simulink model "StorqueV2"  (Simulink 7.5)
settings: Solver=ode45  StartTime=0.0  StopTime=10.0  RelTol=1e-3
undefined symbols (not defined in the file or in its folder): armLength, g, Ixx, Iyy, Izz, KdPhi, KdPsi, KdTheta, KiPhi, KiPsi, KiTheta, KpPhi, KpPsi, KpTheta, mass, PWMMax, PWMMin, PWMPerThrust, tau1, tau2, tau3, tau4
settings Model: Creator=ianohara  LastModifiedBy=ianohara

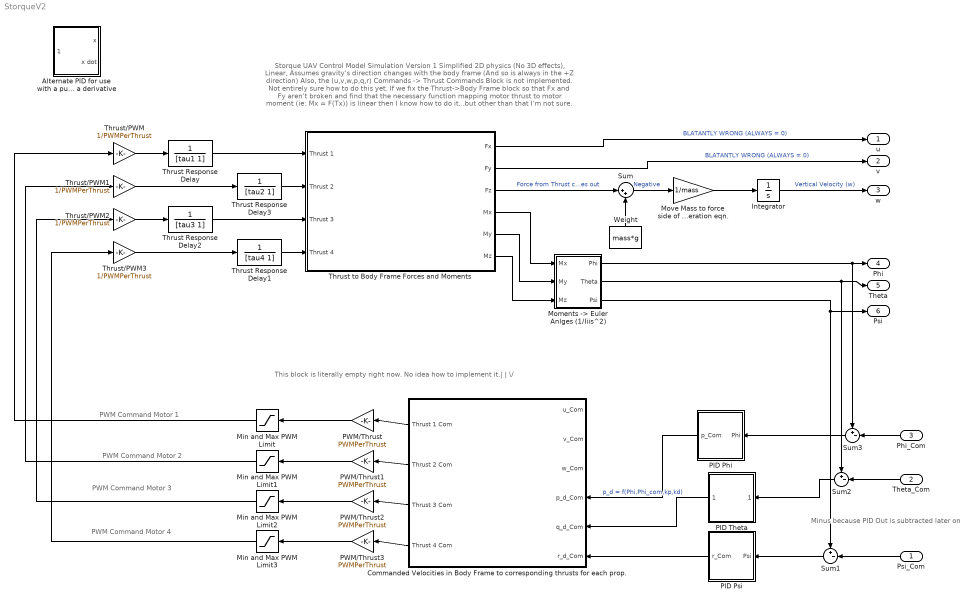
== system StorqueV2 ==
  note: PWM Command Motor 1
  note: PWM Command Motor 2
  note: PWM Command Motor 3
  note: PWM Command Motor 4
  note: This block is literally empty right now.
      | No idea how to implement it.|
      |                                               |
      |                                                \/
  note: Storque UAV Control Model Simulation Version 1
      | Simplified 2D physics (No 3D effects), Linear, Assumes gravity's direction changes with
      | the body frame (And so is always in the +Z direction)
      |
      | Also, the (u,v,w,p,q,r) Commands -> Thrust Commands Block is not implemented.
      | Not entirely sure how to do this yet.  If we fix the Thrust->Body Frame block so that
      | Fx and Fy aren't broken and find that the necessary function mapping motor thrust to motor
      | moment (ie: Mx = F(Tx)) is linear then I know how to do it...but other than that I'm not sure.
  note: Minus because PID
      | Out is subtracted later on
  Psi_Com : Inport  OutDataType=fixdt(1, 16)  OutScaling=2^0
  Theta_Com : Inport  Port=2  OutDataType=fixdt(1, 16)  OutScaling=2^0
  Phi_Com : Inport  Port=3  OutDataType=fixdt(1, 16)  OutScaling=2^0
  Alternate PID for use with a pure rate signal instead of taking a derivative : Subsystem
  Commanded Velocities in Body Frame to corresponding thrusts for each prop. : Subsystem
  Integrator : Integrator
  Min and Max PWM Limit{,1..3} (4 alike) : Saturate  UpperLimit=PWMMax  LowerLimit=PWMMin  OutDataType=fixdt(1, 16)  OutScaling=2^0
  "Moments -> Euler Anlges (1/Iiis^2)" : Subsystem
  Move Mass to force side of acceleration eqn. : Gain  Gain=1/mass  ParameterDataType=fixdt(1, 16)  ParameterScaling=2^0  OutDataType=fixdt(1, 16)  OutScaling=2^0
  PID Phi : Subsystem
  PID Psi : Subsystem
  PID Theta : Subsystem
  PWM/Thrust{,1..3} (4 alike) : Gain  Gain=PWMPerThrust  ParameterDataType=fixdt(1, 16)  ParameterScaling=2^0  OutDataType=fixdt(1, 16)  OutScaling=2^0
  Sum : Sum  Inputs=|++  OutDataType=fixdt(1, 16)  OutScaling=2^0
  Sum1 : Sum  Inputs=+-|  OutDataType=fixdt(1, 16)  OutScaling=2^0
  Sum2 : Sum  Inputs=+-|  OutDataType=fixdt(1, 16)  OutScaling=2^0
  Sum3 : Sum  Inputs=+-|  OutDataType=fixdt(1, 16)  OutScaling=2^0
  Thrust Response Delay : TransferFcn  Denominator=[tau1 1]
  Thrust Response Delay1 : TransferFcn  Denominator=[tau4 1]
  Thrust Response Delay2 : TransferFcn  Denominator=[tau3 1]
  Thrust Response Delay3 : TransferFcn  Denominator=[tau2 1]
  Thrust to Body Frame Forces and Moments : Subsystem  Description=This simulates the body frame reactions of the Storque due to the application of a particular thrust at each of the 4 props.
  Thrust/PWM{,1..3} (4 alike) : Gain  Gain=1/PWMPerThrust  ParameterDataType=fixdt(1, 16)  ParameterScaling=2^0  OutDataType=fixdt(1, 16)  OutScaling=2^0
  Weight : Constant  Value=mass*g  OutDataType=fixdt(1, 16)  OutScaling=2^0
  u : Outport  OutDataType=fixdt(1, 16)  OutScaling=2^0
  v : Outport  Port=2  OutDataType=fixdt(1, 16)  OutScaling=2^0
  w : Outport  Port=3  OutDataType=fixdt(1, 16)  OutScaling=2^0
  Phi : Outport  Port=4  OutDataType=fixdt(1, 16)  OutScaling=2^0
  Theta : Outport  Port=5  OutDataType=fixdt(1, 16)  OutScaling=2^0
  Psi : Outport  Port=6  OutDataType=fixdt(1, 16)  OutScaling=2^0
  wires:
  Thrust to Body Frame Forces and Moments/3(Fz) -> Sum/1  "Force from Thrust comes out                 Negative"
  Weight/1 -> Sum/2
  Sum/1 -> Move Mass to force side of acceleration eqn./1
  Move Mass to force side of acceleration eqn./1 -> Integrator/1
  Integrator/1 -> w/1  "Vertical Velocity (w)"
  Thrust to Body Frame Forces and Moments/6(Mz) -> "Moments -> Euler Anlges (1/Iiis^2)"/3(Mz)
  Thrust to Body Frame Forces and Moments/5(My) -> "Moments -> Euler Anlges (1/Iiis^2)"/2(My)
  Thrust to Body Frame Forces and Moments/4(Mx) -> "Moments -> Euler Anlges (1/Iiis^2)"/1(Mx)
  Thrust to Body Frame Forces and Moments/1(Fx) -> u/1  "BLATANTLY WRONG (ALWAYS = 0)"
  Thrust to Body Frame Forces and Moments/2(Fy) -> v/1  "BLATANTLY WRONG (ALWAYS = 0)"
  "Moments -> Euler Anlges (1/Iiis^2)"/1(Phi) -> Phi/1, Sum3/1
  "Moments -> Euler Anlges (1/Iiis^2)"/2(Theta) -> Theta/1, Sum2/1
  "Moments -> Euler Anlges (1/Iiis^2)"/3(Psi) -> Sum1/1, Psi/1
  Sum1/1 -> PID Psi/1(Psi)
  Sum2/1 -> PID Theta/1(Theta)
  Sum3/1 -> PID Phi/1(Phi)
  Psi_Com/1 -> Sum1/2
  Theta_Com/1 -> Sum2/2
  Phi_Com/1 -> Sum3/2
  Thrust Response Delay/1 -> Thrust to Body Frame Forces and Moments/1(Thrust 1)
  Thrust Response Delay3/1 -> Thrust to Body Frame Forces and Moments/2(Thrust 2)
  Thrust Response Delay2/1 -> Thrust to Body Frame Forces and Moments/3(Thrust 3)
  Thrust Response Delay1/1 -> Thrust to Body Frame Forces and Moments/4(Thrust 4)
  PID Psi/1(r_Com) -> Commanded Velocities in Body Frame to corresponding thrusts for each prop./6(r_d_Com)
  PID Theta/1(q_Com) -> Commanded Velocities in Body Frame to corresponding thrusts for each prop./5(q_d_Com)
  PID Phi/1(p_Com) -> Commanded Velocities in Body Frame to corresponding thrusts for each prop./4(p_d_Com)  "p_d = f(Phi,Phi_com,kp,kd)"
  Commanded Velocities in Body Frame to corresponding thrusts for each prop./1(Thrust 1 Com) -> PWM/Thrust/1
  Commanded Velocities in Body Frame to corresponding thrusts for each prop./2(Thrust 2 Com) -> PWM/Thrust1/1
  Commanded Velocities in Body Frame to corresponding thrusts for each prop./3(Thrust 3 Com) -> PWM/Thrust2/1
  Commanded Velocities in Body Frame to corresponding thrusts for each prop./4(Thrust 4 Com) -> PWM/Thrust3/1
  PWM/Thrust/1 -> Min and Max PWM Limit/1
  PWM/Thrust1/1 -> Min and Max PWM Limit1/1
  PWM/Thrust2/1 -> Min and Max PWM Limit2/1
  PWM/Thrust3/1 -> Min and Max PWM Limit3/1
  Min and Max PWM Limit/1 -> Thrust/PWM/1
  Min and Max PWM Limit1/1 -> Thrust/PWM1/1
  Min and Max PWM Limit2/1 -> Thrust/PWM2/1
  Min and Max PWM Limit3/1 -> Thrust/PWM3/1
  Thrust/PWM3/1 -> Thrust Response Delay1/1
  Thrust/PWM2/1 -> Thrust Response Delay2/1
  Thrust/PWM1/1 -> Thrust Response Delay3/1
  Thrust/PWM/1 -> Thrust Response Delay/1

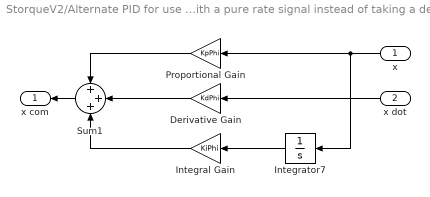
== system StorqueV2/Alternate PID for use with a pure rate signal instead of taking a derivative ==
  x : Inport  OutDataType=fixdt(1, 16)  OutScaling=2^0
  x dot : Inport  Port=2  OutDataType=fixdt(1, 16)  OutScaling=2^0
  Derivative Gain : Gain  Gain=KdPhi  ParameterDataType=fixdt(1, 16)  ParameterScaling=2^0  OutDataType=fixdt(1, 16)  OutScaling=2^0
  Integral Gain : Gain  Gain=KiPhi  ParameterDataType=fixdt(1, 16)  ParameterScaling=2^0  OutDataType=fixdt(1, 16)  OutScaling=2^0
  Integrator7 : Integrator
  Proportional Gain : Gain  Gain=KpPhi  ParameterDataType=fixdt(1, 16)  ParameterScaling=2^0  OutDataType=fixdt(1, 16)  OutScaling=2^0
  Sum1 : Sum  Inputs=+++  OutDataType=fixdt(1, 16)  OutScaling=2^0
  x com : Outport
  wires:
  Integral Gain/1 -> Sum1/3
  Derivative Gain/1 -> Sum1/2
  Proportional Gain/1 -> Sum1/1
  x dot/1 -> Derivative Gain/1
  Integrator7/1 -> Integral Gain/1
  Sum1/1 -> x com/1
  x/1 -> Proportional Gain/1, Integrator7/1

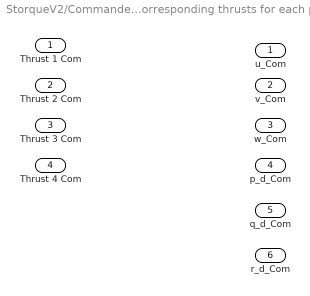
== system StorqueV2/Commanded Velocities in Body Frame to corresponding thrusts for each prop. ==
  u_Com : Inport  OutDataType=fixdt(1, 16)  OutScaling=2^0
  v_Com : Inport  Port=2  OutDataType=fixdt(1, 16)  OutScaling=2^0
  w_Com : Inport  Port=3  OutDataType=fixdt(1, 16)  OutScaling=2^0
  p_d_Com : Inport  Port=4  OutDataType=fixdt(1, 16)  OutScaling=2^0
  q_d_Com : Inport  Port=5  OutDataType=fixdt(1, 16)  OutScaling=2^0
  r_d_Com : Inport  Port=6  OutDataType=fixdt(1, 16)  OutScaling=2^0
  Thrust 1 Com : Outport  OutDataType=fixdt(1, 16)  OutScaling=2^0
  Thrust 2 Com : Outport  Port=2  OutDataType=fixdt(1, 16)  OutScaling=2^0
  Thrust 3 Com : Outport  Port=3  OutDataType=fixdt(1, 16)  OutScaling=2^0
  Thrust 4 Com : Outport  Port=4  OutDataType=fixdt(1, 16)  OutScaling=2^0

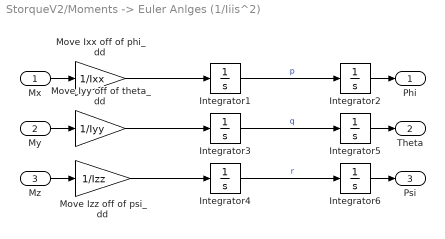
== system StorqueV2/Moments -> Euler Anlges (1/Iiis^2) ==
  Mx : Inport
  My : Inport  Port=2
  Mz : Inport  Port=3
  Integrator{1..6} (6 alike) : Integrator
  Move Ixx off of phi_dd : Gain  Gain=1/Ixx  ParameterDataType=fixdt(1, 16)  ParameterScaling=2^0  OutDataType=fixdt(1, 16)  OutScaling=2^0
  Move Iyy off of theta_dd : Gain  Gain=1/Iyy  ParameterDataType=fixdt(1, 16)  ParameterScaling=2^0  OutDataType=fixdt(1, 16)  OutScaling=2^0
  Move Izz off of psi_dd : Gain  Gain=1/Izz  ParameterDataType=fixdt(1, 16)  ParameterScaling=2^0  OutDataType=fixdt(1, 16)  OutScaling=2^0
  Phi : Outport
  Theta : Outport  Port=2
  Psi : Outport  Port=3
  wires:
  Move Ixx off of phi_dd/1 -> Integrator1/1
  Integrator1/1 -> Integrator2/1  "p"
  Move Iyy off of theta_dd/1 -> Integrator3/1
  Integrator3/1 -> Integrator5/1  "q"
  Move Izz off of psi_dd/1 -> Integrator4/1
  Integrator4/1 -> Integrator6/1  "r"
  Integrator2/1 -> Phi/1
  Mx/1 -> Move Ixx off of phi_dd/1
  Integrator5/1 -> Theta/1
  My/1 -> Move Iyy off of theta_dd/1
  Integrator6/1 -> Psi/1
  Mz/1 -> Move Izz off of psi_dd/1

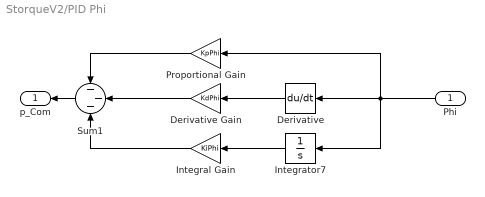
== system StorqueV2/PID Phi ==
  Phi : Inport  OutDataType=fixdt(1, 16)  OutScaling=2^0
  Derivative : Derivative
  Derivative Gain : Gain  Gain=KdPhi  ParameterDataType=fixdt(1, 16)  ParameterScaling=2^0  OutDataType=fixdt(1, 16)  OutScaling=2^0
  Integral Gain : Gain  Gain=KiPhi  ParameterDataType=fixdt(1, 16)  ParameterScaling=2^0  OutDataType=fixdt(1, 16)  OutScaling=2^0
  Integrator7 : Integrator
  Proportional Gain : Gain  Gain=KpPhi  ParameterDataType=fixdt(1, 16)  ParameterScaling=2^0  OutDataType=fixdt(1, 16)  OutScaling=2^0
  Sum1 : Sum  Inputs=---  OutDataType=fixdt(1, 16)  OutScaling=2^0
  p_Com : Outport
  wires:
  Integral Gain/1 -> Sum1/3
  Derivative Gain/1 -> Sum1/2
  Proportional Gain/1 -> Sum1/1
  Derivative/1 -> Derivative Gain/1
  Integrator7/1 -> Integral Gain/1
  Phi/1 -> Derivative/1, Proportional Gain/1, Integrator7/1
  Sum1/1 -> p_Com/1

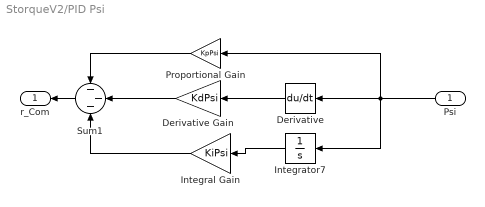
== system StorqueV2/PID Psi ==
  Psi : Inport  OutDataType=fixdt(1, 16)  OutScaling=2^0
  Derivative : Derivative
  Derivative Gain : Gain  Gain=KdPsi  ParameterDataType=fixdt(1, 16)  ParameterScaling=2^0  OutDataType=fixdt(1, 16)  OutScaling=2^0
  Integral Gain : Gain  Gain=KiPsi  ParameterDataType=fixdt(1, 16)  ParameterScaling=2^0  OutDataType=fixdt(1, 16)  OutScaling=2^0
  Integrator7 : Integrator
  Proportional Gain : Gain  Gain=KpPsi  ParameterDataType=fixdt(1, 16)  ParameterScaling=2^0  OutDataType=fixdt(1, 16)  OutScaling=2^0
  Sum1 : Sum  Inputs=---  OutDataType=fixdt(1, 16)  OutScaling=2^0
  r_Com : Outport
  wires:
  Integral Gain/1 -> Sum1/3
  Derivative Gain/1 -> Sum1/2
  Proportional Gain/1 -> Sum1/1
  Derivative/1 -> Derivative Gain/1
  Integrator7/1 -> Integral Gain/1
  Psi/1 -> Derivative/1, Proportional Gain/1, Integrator7/1
  Sum1/1 -> r_Com/1

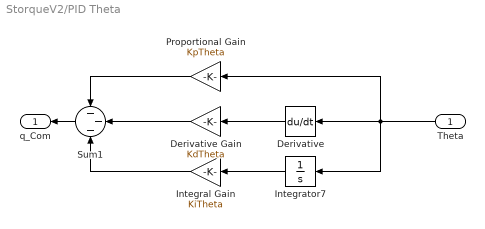
== system StorqueV2/PID Theta ==
  Theta : Inport  OutDataType=fixdt(1, 16)  OutScaling=2^0
  Derivative : Derivative
  Derivative Gain : Gain  Gain=KdTheta  ParameterDataType=fixdt(1, 16)  ParameterScaling=2^0  OutDataType=fixdt(1, 16)  OutScaling=2^0
  Integral Gain : Gain  Gain=KiTheta  ParameterDataType=fixdt(1, 16)  ParameterScaling=2^0  OutDataType=fixdt(1, 16)  OutScaling=2^0
  Integrator7 : Integrator
  Proportional Gain : Gain  Gain=KpTheta  ParameterDataType=fixdt(1, 16)  ParameterScaling=2^0  OutDataType=fixdt(1, 16)  OutScaling=2^0
  Sum1 : Sum  Inputs=---  OutDataType=fixdt(1, 16)  OutScaling=2^0
  q_Com : Outport
  wires:
  Integral Gain/1 -> Sum1/3
  Derivative Gain/1 -> Sum1/2
  Proportional Gain/1 -> Sum1/1
  Derivative/1 -> Derivative Gain/1
  Integrator7/1 -> Integral Gain/1
  Theta/1 -> Derivative/1, Proportional Gain/1, Integrator7/1
  Sum1/1 -> q_Com/1

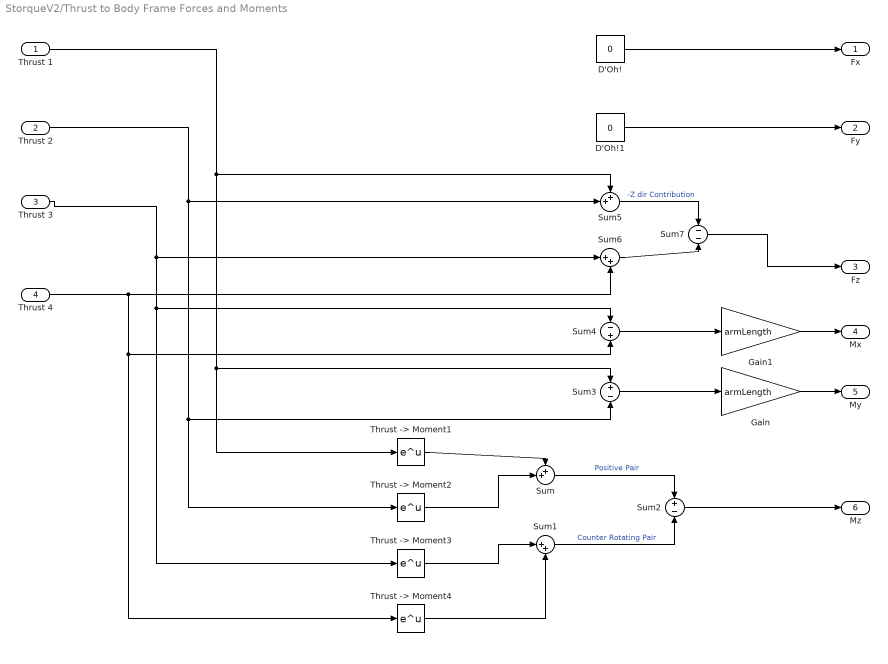
== system StorqueV2/Thrust to Body Frame Forces and Moments ==
  Thrust 1 : Inport  OutDataType=fixdt(1, 16)  OutScaling=2^0
  Thrust 2 : Inport  Port=2  OutDataType=fixdt(1, 16)  OutScaling=2^0
  Thrust 3 : Inport  Port=3  OutDataType=fixdt(1, 16)  OutScaling=2^0
  Thrust 4 : Inport  Port=4  OutDataType=fixdt(1, 16)  OutScaling=2^0
  D'Oh! : Constant  Value=0  OutDataType=fixdt(1, 16)  OutScaling=2^0
  D'Oh!1 : Constant  Value=0  OutDataType=fixdt(1, 16)  OutScaling=2^0
  Gain : Gain  Gain=armLength  ParameterDataType=fixdt(1, 16)  ParameterScaling=2^0  OutDataType=fixdt(1, 16)  OutScaling=2^0
  Gain1 : Gain  Gain=armLength  ParameterDataType=fixdt(1, 16)  ParameterScaling=2^0  OutDataType=fixdt(1, 16)  OutScaling=2^0
  Sum : Sum  Inputs=++|  OutDataType=fixdt(1, 16)  OutScaling=2^0
  Sum1 : Sum  Inputs=|++  OutDataType=fixdt(1, 16)  OutScaling=2^0
  Sum2 : Sum  Inputs=+|-  OutDataType=fixdt(1, 16)  OutScaling=2^0
  Sum3 : Sum  Inputs=+|-  OutDataType=fixdt(1, 16)  OutScaling=2^0
  Sum4 : Sum  Inputs=-|+  OutDataType=fixdt(1, 16)  OutScaling=2^0
  Sum5 : Sum  Inputs=++|  OutDataType=fixdt(1, 16)  OutScaling=2^0
  Sum6 : Sum  Inputs=|++  OutDataType=fixdt(1, 16)  OutScaling=2^0
  Sum7 : Sum  Inputs=-|-  OutDataType=fixdt(1, 16)  OutScaling=2^0
  Thrust -> Moment{1..4} (4 alike) : Math  OutDataType=fixdt(1, 16)  OutScaling=2^0  SaturateOnIntegerOverflow=on
  Fx : Outport  OutDataType=fixdt(1, 16)  OutScaling=2^0
  Fy : Outport  Port=2  OutDataType=fixdt(1, 16)  OutScaling=2^0
  Fz : Outport  Port=3  OutDataType=fixdt(1, 16)  OutScaling=2^0
  Mx : Outport  Port=4  OutDataType=fixdt(1, 16)  OutScaling=2^0
  My : Outport  Port=5  OutDataType=fixdt(1, 16)  OutScaling=2^0
  Mz : Outport  Port=6  OutDataType=fixdt(1, 16)  OutScaling=2^0
  wires:
  D'Oh!/1 -> Fx/1
  D'Oh!1/1 -> Fy/1
  Sum7/1 -> Fz/1
  Sum6/1 -> Sum7/2
  Sum5/1 -> Sum7/1  "-Z dir Contribution"
  Gain1/1 -> Mx/1
  Sum4/1 -> Gain1/1
  Gain/1 -> My/1
  Sum3/1 -> Gain/1
  Sum2/1 -> Mz/1
  "Thrust -> Moment4"/1 -> Sum1/2
  "Thrust -> Moment3"/1 -> Sum1/1
  "Thrust -> Moment2"/1 -> Sum/2
  "Thrust -> Moment1"/1 -> Sum/1
  Thrust 4/1 -> Sum6/2, Sum4/2, "Thrust -> Moment4"/1
  Thrust 3/1 -> Sum6/1, Sum4/1, "Thrust -> Moment3"/1
  Thrust 2/1 -> Sum5/2, Sum3/2, "Thrust -> Moment2"/1
  Thrust 1/1 -> Sum5/1, "Thrust -> Moment1"/1, Sum3/1
  Sum1/1 -> Sum2/2  "Counter Rotating Pair"
  Sum/1 -> Sum2/1  "Positive Pair"
